simulink model "MPC_simulation"  (R2019b)
settings: Solver=FixedStepDiscrete  StartTime=0.0  StopTime=20  FixedStep=0.01  RelTol=1e-3
InitFcn:
  | Np = 10; Nc = 10;
settings Model: Creator=seokhun  LastModifiedBy=seokhun
settings DebuggingCC: UnderSpecifiedDimensionMsg=warning

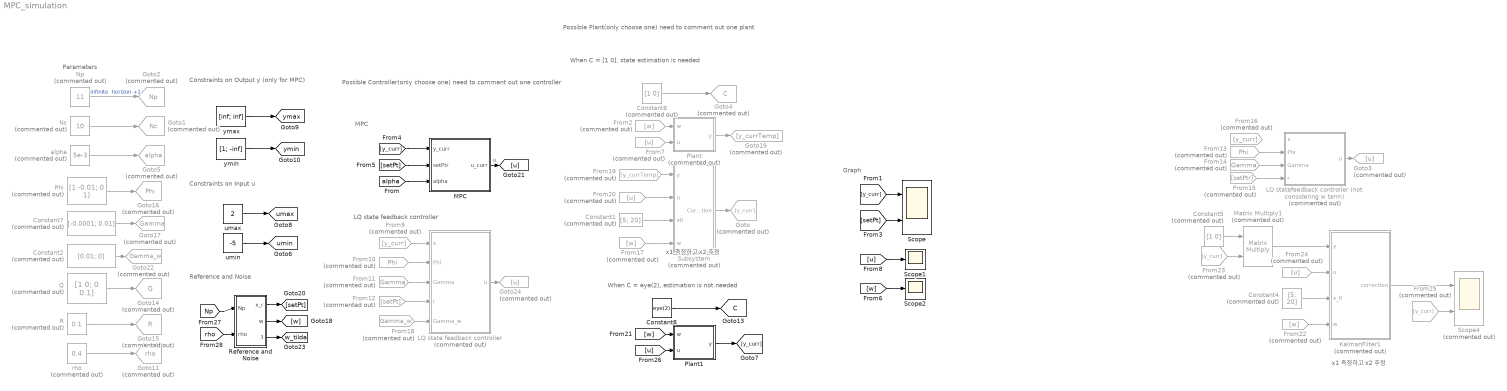
== system MPC_simulation ==
  note: Constraints on Input u
  note: LQ state feedback controller
  note: MPC
  note: Possible Plant(only choose one)
      | need to comment out one plant
  note: When C = eye(2), estimation is not needed
  note: When C = [1 0], state estimation is needed
  note: x1 측정하고 x2 추정
  note: x1 측정하고 x2 추정
  note: Possible Controller(only choose one)
      | need to comment out one controller
  note: Reference and Noise
  note: Parameters
  note: Graph
  note: Constraints on Output y
      | (only for MPC)
  Constant1 : Constant  Commented=on  Value=[5; 20]
  Constant2 : Constant  Commented=on  Value=[0.01; 0]  VectorParams1D=off
  Constant4 : Constant  Commented=on  Value=[5; 20]
  Constant5 : Constant  Commented=on  Value=[1 0]  VectorParams1D=off
  Constant6 : Constant  Commented=on  Value=[1 0]  VectorParams1D=off
  Constant7 : Constant  Commented=on  Value=[-0.0001; 0.01]  VectorParams1D=off
  Constant8 : Constant  Value=eye(2)  VectorParams1D=off
  From10 : From  Commented=on  GotoTag=Phi  TagVisibility=global
  From11 : From  Commented=on  GotoTag=Gamma  TagVisibility=global
  From12 : From  Commented=on  GotoTag=setPt
  From13 : From  Commented=on  GotoTag=Phi  TagVisibility=global
  From14 : From  Commented=on  GotoTag=Gamma  TagVisibility=global
  From15 : From  Commented=on  GotoTag=setPtr
  From{9,16,23,25} (4 alike) : From  Commented=on  GotoTag=y_curr
  From17 : From  Commented=on  GotoTag=w
  From18 : From  Commented=on  GotoTag=Gamma_w  TagVisibility=global
  From19 : From  Commented=on  GotoTag=y_currTemp
  From2 : From  Commented=on  GotoTag=w
  From20 : From  Commented=on  GotoTag=u
  From22 : From  Commented=on  GotoTag=w
  From24 : From  Commented=on  GotoTag=u
  From7 : From  Commented=on  GotoTag=u
  Goto : Goto  Commented=on  GotoTag=y_curr
  Goto1 : Goto  Commented=on  GotoTag=Nc  TagVisibility=global
  Goto11 : Goto  Commented=on  GotoTag=rho  TagVisibility=global
  Goto14 : Goto  Commented=on  GotoTag=Q  TagVisibility=global
  Goto15 : Goto  Commented=on  GotoTag=R  TagVisibility=global
  Goto16 : Goto  Commented=on  GotoTag=Phi  TagVisibility=global
  Goto17 : Goto  Commented=on  GotoTag=Gamma  TagVisibility=global
  Goto19 : Goto  Commented=on  GotoTag=y_currTemp
  Goto2 : Goto  Commented=on  GotoTag=Np  TagVisibility=global
  Goto22 : Goto  Commented=on  GotoTag=Gamma_w  TagVisibility=global
  Goto24 : Goto  Commented=on  GotoTag=u
  Goto3 : Goto  Commented=on  GotoTag=u
  Goto4 : Goto  Commented=on  GotoTag=C  TagVisibility=global
  Goto5 : Goto  Commented=on  GotoTag=alpha  TagVisibility=global
  KalmanFilter1 : MATLAB Function  Commented=on  TreatAsAtomicUnit=on
  LQ state feedback controller : Subsystem  Commented=on
  LQ statefeedback controller (not considering w term) : Subsystem  Commented=on
  MPC : Subsystem
  Matrix Multiply1 : Product  Commented=on  Multiplication=Matrix(*)
  Nc : Constant  Commented=on  Value=10
  Np : Constant  Commented=on  Value=11
  Phi : Constant  Commented=on  Value=[1 -0.01; 0 1]
  Plant : Subsystem  Commented=on
  Plant1 : Subsystem
  Q : Constant  Commented=on  Value=[1 0; 0 0.1]
  R : Constant  Commented=on  Value=0.1  VectorParams1D=off
  Reference and Noise : Subsystem
  Scope : Scope  NumInputPorts=2
  Scope1 : Scope
  Scope2 : Scope
  Scope4 : Scope  Commented=on  NumInputPorts=2
  Subsystem : Subsystem  Commented=on
  alpha : Constant  Commented=on  Value=5e-3
  rho : Constant  Commented=on  Value=0.4
  umax : Constant  Value=2
  umin : Constant  Value=-5
  ymax : Constant  Value=[inf; inf]  VectorParams1D=off
  ymin : Constant  Value=[1; -inf]  VectorParams1D=off
  tag scope: C=global, umax=global, umin=global, w_tilda=global, ymax=global, ymin=global
  wires:
  alpha/1 -> Goto5/1
  Nc/1 -> Goto1/1
  Np/1 -> Goto2/1  "infinite  horizon +1"
  R/1 -> Goto15/1
  Constant8/1 -> [C]
  Phi/1 -> Goto16/1
  Constant7/1 -> Goto17/1
  Q/1 -> Goto14/1
  Reference and Noise/1(x_r) -> [setPt]
  Plant/1(y) -> Goto19/1
  From2/1 -> Plant/1(w)
  [y_curr] -> Scope/1
  [setPt] -> Scope/2
  Reference and Noise/2(w) -> [w]
  [y_curr] -> MPC/1(y_curr)
  [setPt] -> MPC/2(setPtr)
  [alpha] -> MPC/3(alpha)
  [w] -> Scope2/1
  MPC/1(u_curr) -> [u]  "u"
  From7/1 -> Plant/2(u)
  [u] -> Scope1/1
  Constant2/1 -> Goto22/1
  Reference and Noise/3(w_tilda) -> [w_tilda]
  From9/1 -> LQ state feedback controller/1(x)
  From10/1 -> LQ state feedback controller/2(Phi)
  From11/1 -> LQ state feedback controller/3(Gamma)
  From12/1 -> LQ state feedback controller/4(r)
  LQ state feedback controller/1(u) -> Goto24/1
  LQ statefeedback controller (not considering w term)/1(u) -> Goto3/1
  From15/1 -> LQ statefeedback controller (not considering w term)/4(r)
  From14/1 -> LQ statefeedback controller (not considering w term)/3(Gamma)
  From13/1 -> LQ statefeedback controller (not considering w term)/2(Phi)
  From18/1 -> LQ state feedback controller/5(Gamma_w)
  From25/1 -> Scope4/2
  KalmanFilter1/1(correction) -> Scope4/1
  Constant5/1 -> Matrix Multiply1/1
  Matrix Multiply1/1 -> KalmanFilter1/1(y)
  From23/1 -> Matrix Multiply1/2
  From24/1 -> KalmanFilter1/2(u)
  Constant4/1 -> KalmanFilter1/3(x_0)
  From22/1 -> KalmanFilter1/4(w)
  Constant6/1 -> Goto4/1
  [u] -> Plant1/2(u)
  [w] -> Plant1/1(w)
  Plant1/1(y) -> [y_curr]
  From19/1 -> Subsystem/1(y)
  From20/1 -> Subsystem/2(u)
  Constant1/1 -> Subsystem/3(x0)
  From17/1 -> Subsystem/4(w)
  Subsystem/1(Correction) -> Goto/1
  [Np] -> Reference and Noise/1(Np)
  umax/1 -> [umax]
  umin/1 -> [umin]
  ymax/1 -> [ymax]
  ymin/1 -> [ymin]
  [rho] -> Reference and Noise/2(rho)
  rho/1 -> Goto11/1

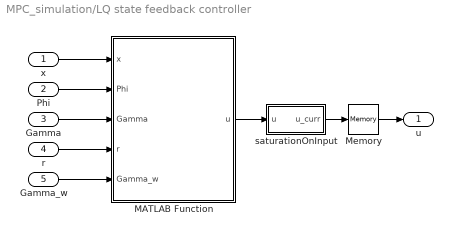
== system MPC_simulation/LQ state feedback controller ==
  x : Inport
  Phi : Inport  Port=2
  Gamma : Inport  Port=3
  r : Inport  Port=4
  Gamma_w : Inport  Port=5
  MATLAB Function : MATLAB Function  TreatAsAtomicUnit=on
  Memory : Memory
  saturationOnInput : Subsystem
  u : Outport
  wires:
  x/1 -> MATLAB Function/1(x)
  saturationOnInput/1(u_curr) -> Memory/1
  Gamma/1 -> MATLAB Function/3(Gamma)
  Memory/1 -> u/1
  r/1 -> MATLAB Function/4(r)
  Phi/1 -> MATLAB Function/2(Phi)
  Gamma_w/1 -> MATLAB Function/5(Gamma_w)
  MATLAB Function/1(u) -> saturationOnInput/1(u)

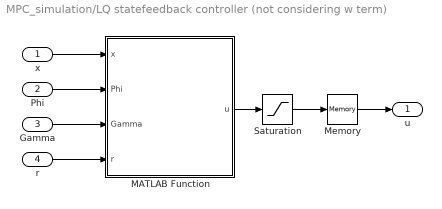
== system MPC_simulation/LQ statefeedback controller (not considering w term) ==
  x : Inport
  Phi : Inport  Port=2
  Gamma : Inport  Port=3
  r : Inport  Port=4
  MATLAB Function : MATLAB Function  TreatAsAtomicUnit=on
  Memory : Memory
  Saturation : Saturate  UpperLimit=2  LowerLimit=-5
  u : Outport
  wires:
  Phi/1 -> MATLAB Function/2(Phi)
  r/1 -> MATLAB Function/4(r)
  Memory/1 -> u/1
  Gamma/1 -> MATLAB Function/3(Gamma)
  Saturation/1 -> Memory/1
  MATLAB Function/1(u) -> Saturation/1
  x/1 -> MATLAB Function/1(x)

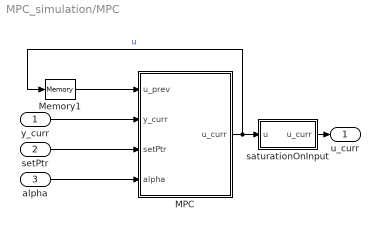
== system MPC_simulation/MPC ==
  y_curr : Inport
  setPtr : Inport  Port=2
  alpha : Inport  Port=3
  MPC : Subsystem
  Memory1 : Memory
  saturationOnInput : Subsystem
  u_curr : Outport
  wires:
  MPC/1(u_curr) -> saturationOnInput/1(u), Memory1/1  "u"
  y_curr/1 -> MPC/2(y_curr)
  alpha/1 -> MPC/4(alpha)
  Memory1/1 -> MPC/1(u_prev)
  setPtr/1 -> MPC/3(setPtr)
  saturationOnInput/1(u_curr) -> u_curr/1

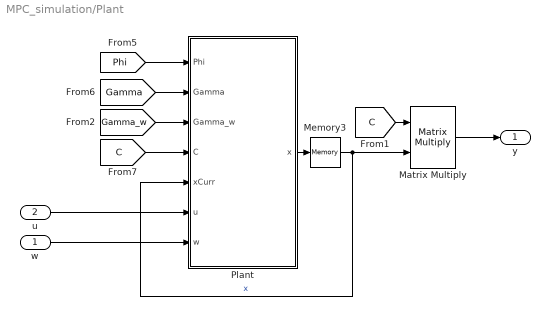
== system MPC_simulation/Plant ==
  w : Inport
  u : Inport  Port=2
  Matrix Multiply : Product  Multiplication=Matrix(*)
  Memory3 : Memory  InitialCondition=[5; 20]
  Plant : MATLAB Function  TreatAsAtomicUnit=on
  y : Outport
  wires:
  Memory3/1 -> Plant/5(xCurr), Matrix Multiply/2  "x"
  u/1 -> Plant/6(u)
  [Gamma] -> Plant/2(Gamma)
  w/1 -> Plant/7(w)
  Plant/1(x) -> Memory3/1
  [C] -> Matrix Multiply/1
  [Phi] -> Plant/1(Phi)
  [C] -> Plant/4(C)
  Matrix Multiply/1 -> y/1
  [Gamma_w] -> Plant/3(Gamma_w)

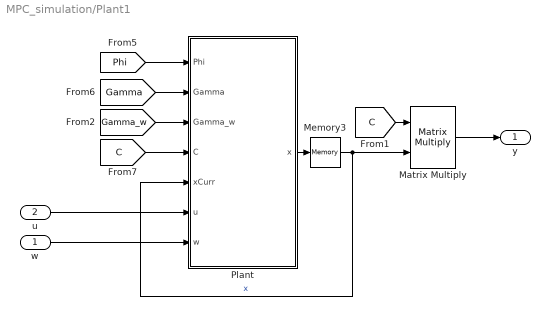
== system MPC_simulation/Plant1 ==
  w : Inport
  u : Inport  Port=2
  Matrix Multiply : Product  Multiplication=Matrix(*)
  Memory3 : Memory  InitialCondition=[5; 20]
  Plant : MATLAB Function  TreatAsAtomicUnit=on
  y : Outport
  wires:
  [Gamma_w] -> Plant/3(Gamma_w)
  Matrix Multiply/1 -> y/1
  [C] -> Plant/4(C)
  [Phi] -> Plant/1(Phi)
  [C] -> Matrix Multiply/1
  Plant/1(x) -> Memory3/1
  w/1 -> Plant/7(w)
  [Gamma] -> Plant/2(Gamma)
  u/1 -> Plant/6(u)
  Memory3/1 -> Matrix Multiply/2, Plant/5(xCurr)  "x"

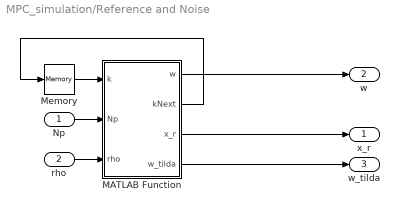
== system MPC_simulation/Reference and Noise ==
  Np : Inport
  rho : Inport  Port=2
  MATLAB Function : MATLAB Function  TreatAsAtomicUnit=on
  Memory : Memory
  x_r : Outport
  w : Outport  Port=2
  w_tilda : Outport  Port=3
  wires:
  MATLAB Function/2(kNext) -> Memory/1
  Memory/1 -> MATLAB Function/1(k)
  MATLAB Function/3(x_r) -> x_r/1
  MATLAB Function/1(w) -> w/1
  MATLAB Function/4(w_tilda) -> w_tilda/1
  Np/1 -> MATLAB Function/2(Np)
  rho/1 -> MATLAB Function/3(rho)

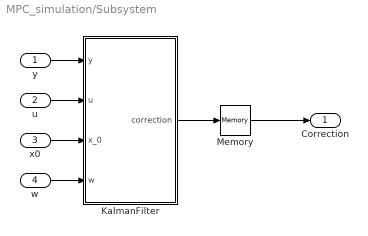
== system MPC_simulation/Subsystem ==
  y : Inport
  u : Inport  Port=2
  x0 : Inport  Port=3
  w : Inport  Port=4
  KalmanFilter : MATLAB Function  TreatAsAtomicUnit=on
  Memory : Memory  InitialCondition=[5; 20]
  Correction : Outport
  wires:
  KalmanFilter/1(correction) -> Memory/1
  x0/1 -> KalmanFilter/3(x_0)
  u/1 -> KalmanFilter/2(u)
  w/1 -> KalmanFilter/4(w)
  y/1 -> KalmanFilter/1(y)
  Memory/1 -> Correction/1

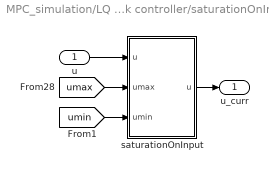
== system MPC_simulation/LQ state feedback controller/saturationOnInput ==
  u : Inport
  saturationOnInput : MATLAB Function  TreatAsAtomicUnit=on
  u_curr : Outport
  wires:
  u/1 -> saturationOnInput/1("u ")
  saturationOnInput/1(u) -> u_curr/1
  [umax] -> saturationOnInput/2(umax)
  [umin] -> saturationOnInput/3(umin)

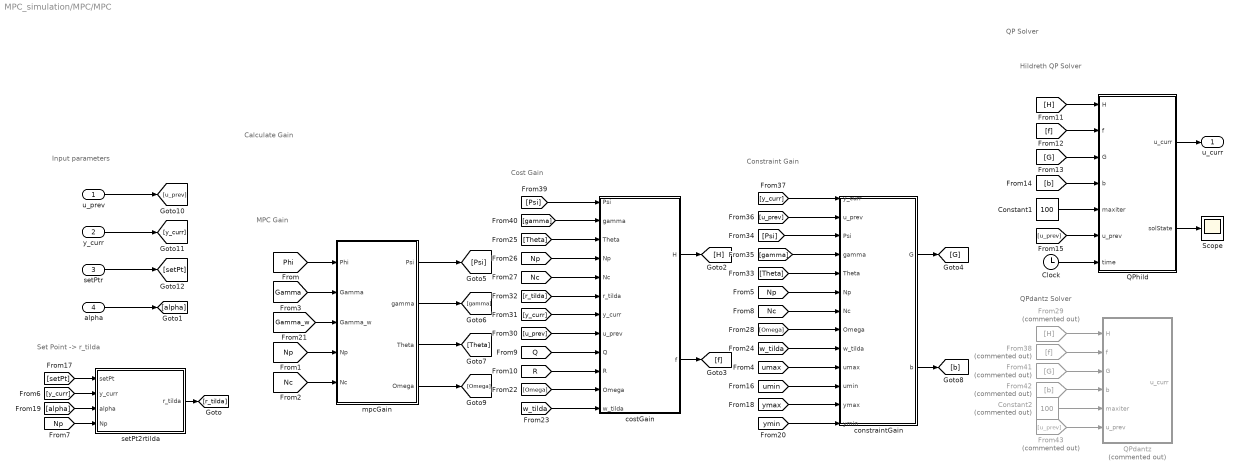
== system MPC_simulation/MPC/MPC ==
  note: QPdantz Solver
  note: Hildreth QP Solver
  note: QP Solver
  note: Set Point -> r_tilda
  note: Cost Gain
  note: Constraint Gain
  note: MPC Gain
  note: Calculate Gain
  note: Input parameters
  u_prev : Inport
  y_curr : Inport  Port=2
  setPtr : Inport  Port=3
  alpha : Inport  Port=4
  Clock : Clock
  Constant1 : Constant  Value=100
  Constant2 : Constant  Commented=on  Value=100
  From29 : From  Commented=on  GotoTag=H
  From38 : From  Commented=on  GotoTag=f
  From41 : From  Commented=on  GotoTag=G
  From42 : From  Commented=on  GotoTag=b
  From43 : From  Commented=on  GotoTag=u_prev
  QPdantz : MATLAB Function  Commented=on  TreatAsAtomicUnit=on
  QPhild : MATLAB Function  TreatAsAtomicUnit=on
  Scope : Scope
  constraintGain : MATLAB Function  TreatAsAtomicUnit=on
  costGain : MATLAB Function  TreatAsAtomicUnit=on
  mpcGain : MATLAB Function  TreatAsAtomicUnit=on
  setPt2rtilda : MATLAB Function  TreatAsAtomicUnit=on
  u_curr : Outport
  wires:
  [Phi] -> mpcGain/1(Phi)
  [Np] -> mpcGain/4(Np)
  mpcGain/1(Psi) -> [Psi]
  [setPt] -> setPt2rtilda/1(setPt)
  u_prev/1 -> [u_prev]
  [Gamma] -> mpcGain/2(Gamma)
  mpcGain/3(Theta) -> [Theta]
  mpcGain/2(gamma) -> [gamma]
  setPtr/1 -> [setPt]
  y_curr/1 -> [y_curr]
  setPt2rtilda/1(r_tilda) -> [r_tilda]
  [y_curr] -> setPt2rtilda/2(y_curr)
  [Np] -> setPt2rtilda/4(Np)
  [alpha] -> setPt2rtilda/3(alpha)
  alpha/1 -> [alpha]
  [Nc] -> mpcGain/5(Nc)
  [Psi] -> constraintGain/3(Psi)
  [u_prev] -> constraintGain/2(u_prev)
  [y_curr] -> constraintGain/1(y_curr)
  [Theta] -> constraintGain/5(Theta)
  [gamma] -> constraintGain/4(gamma)
  [r_tilda] -> costGain/6(r_tilda)
  [u_prev] -> costGain/8(u_prev)
  [Psi] -> costGain/1(Psi)
  [Np] -> costGain/4(Np)
  [y_curr] -> costGain/7(y_curr)
  [Theta] -> costGain/3(Theta)
  [gamma] -> costGain/2(gamma)
  Constant1/1 -> QPhild/5(maxiter)
  [Nc] -> costGain/5(Nc)
  [Np] -> constraintGain/6(Np)
  [Nc] -> constraintGain/7(Nc)
  [Q] -> costGain/9(Q)
  [R] -> costGain/10(R)
  costGain/1(H) -> [H]
  costGain/2(f) -> [f]
  constraintGain/1(G) -> [G]
  constraintGain/2(b) -> [b]
  [H] -> QPhild/1(H)
  [f] -> QPhild/2(f)
  [G] -> QPhild/3(G)
  [b] -> QPhild/4(b)
  [u_prev] -> QPhild/6(u_prev)
  [Gamma_w] -> mpcGain/3(Gamma_w)
  mpcGain/4(Omega) -> [Omega]
  [Omega] -> costGain/11(Omega)
  [w_tilda] -> costGain/12(w_tilda)
  [w_tilda] -> constraintGain/9(w_tilda)
  [Omega] -> constraintGain/8(Omega)
  From42/1 -> QPdantz/4(b)
  From41/1 -> QPdantz/3(G)
  From38/1 -> QPdantz/2(f)
  From29/1 -> QPdantz/1(H)
  Constant2/1 -> QPdantz/5(maxiter)
  From43/1 -> QPdantz/6(u_prev)
  QPhild/1(u_curr) -> u_curr/1
  Clock/1 -> QPhild/7(time)
  QPhild/2(solState) -> Scope/1
  [umax] -> constraintGain/10(umax)
  [umin] -> constraintGain/11(umin)
  [ymax] -> constraintGain/12(ymax)
  [ymin] -> constraintGain/13(ymin)

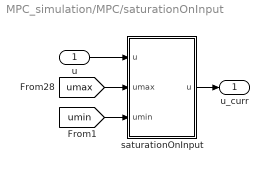
== system MPC_simulation/MPC/saturationOnInput ==
  u : Inport
  saturationOnInput : MATLAB Function  TreatAsAtomicUnit=on
  u_curr : Outport
  wires:
  u/1 -> saturationOnInput/1("u ")
  saturationOnInput/1(u) -> u_curr/1
  [umax] -> saturationOnInput/2(umax)
  [umin] -> saturationOnInput/3(umin)

== matlab function MPC_simulation/MPC/MPC/mpcGain ==
  data: Phi input; Psi output; Gamma input; Gamma_w input; Np input; gamma output; Theta output; Nc input; Omega output
function [Psi, gamma, Theta, Omega] = mpcGain(Phi, Gamma, Gamma_w, Np, Nc)
%%% x(k+1) = Phi*x(k) + Gamma*u(k)
%%% y(k) = C*x(k)

persistent first Psi_y gamma_y Theta_y Omega_y

% Np = 21; Nc = 10;
Np = 11; Nc = 10;
if isempty(first)
    C = eye(2);
    first = 1;    
    %%%%% Find Psi_x, gamma_x, Theta_x and Omega_x
    %%% Psi_x
    [nx, ~] = size(Phi);
    Psi_x = zeros(nx*Np, nx);
    Psi_x(1:nx, :) = eye(nx);
    for i=2:Np    
        Psi_x(nx*(i-1)+1:nx*i, :) = Psi_x(nx*(i-2)+1:nx*(i-1), :)*Phi;
    end

    %%% gamma_x
    [~, nu] = size(Gamma);
    gamma_x = zeros(nx*Np, nu);
    temp = Gamma;
    tempSum = Gamma;
    for i=2:Np
        gamma_x(nx*(i-1)+1:nx*i, :) = tempSum;
        temp = Phi*temp;
        tempSum = tempSum + temp;
    end

    % gamma_xx = [zeros(nx,nu); Gamma; Phi*Gamma+Gamma; Phi^2*Gamma+Phi*Gamma+Gamma]

    %%% Theta_x
    Theta_x = zeros(nx*Np, nu*Nc);
    for j=1:Nc
        if nu == 1
            Theta_x(nx*(j-1)+1:end, j) = gamma_x(1:nx*Np-nx*(j-1), :);
        else
           Theta_x(nx*(j-1)+1:end, nu*(j-1)+1:nu*j) = gamma_x(1:nx*Np-nx*(j-1), :);
        end
    end
    
    %%% Omega_x
    [~, nw] = size(Gamma_w);
    Omega_x = zeros(nx*Np, nw*Np);
    vec = zeros(nx*Np, nw);
    for i=2:Np
        vec(nx*(i-1)+1:nx*i, :) = Psi_x(nx*(i-2)+1:nx*(i-1), :)*Gamma_w;
    end
    for i=1:Np
        if nw == 1
            Omega_x(nx*(i-1)+1:end, i) = vec(1:nx*Np-nx*(i-1), :);
        else        
            Omega_x(nx*(i-1)+1:end, nw*(i-1)+1:nw*i) = vec(1:nx*Np-nx*(i-1), :);
        end
    end
    
    %%%%% Find Psi_x, gamma_x, Theta_x and Omega_x

    %%%%% Find Psi_y, gamma_y, Theta_y and Omega_y
    %%%%% which is equal Psi, gamma, Theta and Omega respectively
    [ny, ~] = size(C);
    C_tilda = zeros(ny*Np, nx*Np);
    for i=1:Np
        if ny == 1            
            C_tilda(i, nx*(i-1)+1:nx*i) = C;
        else
            C_tilda(ny*(i-1)+1:ny*i, nx*(i-1)+1:nx*i) = C;
        end
    end
    Psi_y = C_tilda*Psi_x*C'*(C*C')^-1;
    gamma_y = C_tilda*gamma_x;
    Theta_y = C_tilda*Theta_x;    
    Omega_y = C_tilda*Omega_x;
    %%%%% Find Psi_y, gamma_y, Theta_y and Omega_y
    %%%%% which is equal Psi, gamma, Theta and Omega respectively
end

Psi = Psi_y;
gamma = gamma_y;
Theta = Theta_y;
Omega = Omega_y;

== matlab function MPC_simulation/Plant/Plant ==
  data: Phi input; Gamma input; Gamma_w input; C input; xCurr input; u input; x output; w input
function x  = plant(Phi, Gamma, Gamma_w, C, xCurr, u, w)
% Phi = [1 0.01; 0 1];
% Gamma = [-0.0001; -0.01];
% C = eye(2);

% xNext = Phi*xCurr + Gamma*u; % x(k+1) = Phi*x(k) + gamma2*u(k)
xNext = Phi*xCurr + Gamma*u + Gamma_w*w; % x(k+1) = Phi*x(k) + gamma2*u(k)
x = xNext;
end

== matlab function MPC_simulation/LQ state feedback controller/MATLAB Function ==
  data: x input; Phi input; Gamma input; r input; Gamma_w input; u output
function u = LQcontroller(x, Phi, Gamma, r, Gamma_w)
persistent first leftInv a b nx 
if isempty(first)
    first = 1;
    a = 1; b = 0.1;
    Czx = [a 0; 0 b]; Dzu = [0; 0];
    A = [eye(2)-Phi Gamma; -Czx Dzu];
    [nx, ~] = size(Phi);
    leftInv = (A'*A)^-1*A';
%     xeq = zeros(nx,1); xeq(:) = -p(1:nx); 
%     ueq = zeros(size(Gamma,2)); ueq(:) = p(nx+1:end);
end

% a = 1;  b = 0.1; Czx = [a 0; 0 b];
% Dzu = [0; 0];
% rho = 0.1;
% Q = Czx'*Czx; R = Dzu'*Dzu+rho; N = Czx'*Dzu;
% Phi = [1 -0.01; 0 1]; Gamma = [-0.0001; 0.01];
% [K, ~, ~] = dlqr(Phi, Gamma, Q, R, N);
K = [-3.122453376782691,2.502849098184925];

r(1) = r(1)*a; r(2) = r(2)*b;
w = 20;
q = [-Gamma_w*w; r];
p = leftInv*q; % Ap = q

xeq = zeros(nx,1); xeq(:) = -p(1:nx);
ueq = zeros(size(Gamma,2)); ueq(:) = p(nx+1:end);
u = zeros(size(Gamma,2));
u(:) = -K*(x-xeq) + ueq;
end

== matlab function MPC_simulation/LQ statefeedback controller (not considering w term)/MATLAB Function ==
  data: x input; u output; Phi input; Gamma input; r input
function u = LQcontroller(x, Phi, Gamma, r)
persistent first leftInv a b nx 
if isempty(first)
    first = 1;
    a = 1; b = 0.1;
    Czx = [a 0; 0 b]; Dzu = [0; 0];
    A = [eye(2)-Phi Gamma; -Czx Dzu];
    [nx, ~] = size(Phi);
    leftInv = (A'*A)^-1*A';
end

r(1) = r(1)*a; r(2) = r(2)*b;

q = [zeros(nx,1); r];
p = leftInv*q; % Ap = q 
xeq = zeros(nx,1); xeq(:) = -p(1:nx); 
ueq = zeros(size(Gamma,2)); ueq(:) = p(nx+1:end);

% a = 1;  b = 0.1; G = [a 0; 0 b];
% H = [0; 0];
% rho = 0.1;
% Q = G'*G; R = H'*H+rho; N = G'*H;
% Phi = [1 -0.01; 0 1]; Gamma = [-0.0001; 0.01];
% [K, ~, ~] = dlqr(Phi, Gamma, Q, R, N);
K = [-3.122453376782691,2.502849098184925];


u = zeros(size(Gamma,2));
u(:) = -K*(x-xeq) + ueq;
end

== matlab function MPC_simulation/MPC/MPC/setPt2rtilda ==
  data: setPt input; r_tilda output; y_curr input; alpha input; Np input
function r_tilda = set_pt2r_tilda(setPt, y_curr, alpha, Np)
%%% r_tilda = y_r_tilda(set-point) + r_e_tilda
%%% where r_e(k+i) = y_e(k)*exp(-alpha*i)

Np = 11;
% Np = 21;
[ny, ~] = size(y_curr);
r_tilda = zeros(ny*Np,1);

y_e = y_curr - setPt;

for i=1:Np
    r_tilda(ny*(i-1)+1:ny*i) = setPt + y_e * exp(-alpha*(i-1));
end

== matlab function MPC_simulation/Reference and Noise/MATLAB Function ==
  data: k input; w output; kNext output; x_r output; w_tilda output; Np input; rho input
function [w, kNext, x_r, w_tilda] = makeNoise(k, Np, rho)

delta_k = 25;

x1_r = 5;
x2_r = noise(max(1, k-delta_k), rho);
x_r = [x1_r; x2_r];

w = noise(k, rho);

w_tilda = make_w_tilda(k, Np, rho);

kNext = k + 1;

end

function w = noise(k, rho)

% rho = 0.4;
w0 = 20; ks = 500; kf = ks + 200; 
w = w0*(1-rho*(sin(pi*(min(max(0,k-ks),kf-ks)/(kf-ks)))^2));

end

function w_tilda = make_w_tilda(k, Np, rho)
Np = 11; %%%%%%%%%%%%%%%%%%%%%%
% Np = 21; %%%%%%%%%%%%%%%%%%%%%%
w_tilda = zeros(Np,1);
for i=1:Np
    w_tilda(i) = noise(k+i-1, rho);
end
end

== matlab function MPC_simulation/MPC/MPC/QPdantz ==
  data: H input size=[10, 10]; u_curr output size=1; f input size=[10, 1]; G input size=[84, 10]; b input size=[84, 1]; maxiter input size=1; u_prev input size=1
function u_curr = QPdantzSolver(H, f, G, b, maxiter, u_prev)
nx = 2; Np = 11;
Nc = 10; nu = 1;

delta_u_tilda_umin = -5*ones(nu*Nc,1);

delta_u_tilda = zeros(Nc*nu, 1);
[delta_u_tilda(:), ~, ~] = qpdantzMy(H, f, G, b, delta_u_tilda_umin, maxiter);
% [delta_u_tilda(:), ~, ~] = quadprog(H, f, G, b);

u_curr = zeros(nu,1); 
u_curr(:) = delta_u_tilda(1) + u_prev;
end


function [xopt,lambda,how] = qpdantzMy(H,f,A,b,xmin,maxiter)
%QPDANTZ command will be removed in a future release.  If you have
%   Optimization Toolbox, replace "qpdantz" with "quadprog" command. 
%
% QPDANTZ solves a quadratic program using an active set method.
%
%   [x,lambda,status]=QPDANTZ(H,f,A,b,xmin,maxiter) solves the quadratic
%   programming problem:
%
%     min 0.5*x'Hx + f'x   subject to:  Ax <= b, x >= xmin
%      x
%
%   where:
%        x = the optimal solution vector.
%   lambda = the dual variables (Lagrange multipliers) at the solution.
%   status = 'feasible' if x satisfies the constraints
%          = 'infeasible' if no feasible x could be found
%          = 'unreliable' if maximum number of iterations is exceeded.

%   Author: A. Bemporad
%   Copyright 1986-2011 The MathWorks, Inc.

narginchk(4,6);

if nargin<5 || isempty(xmin)
    xmin=-1e3*ones(size(f(:)));
%     ctrlMsgUtils.warning('MPC:computation:AssumeXMin');    
end

if nargin<6,
    maxiter=200;
end
if maxiter<1,
%     ctrlMsgUtils.error('MPC:computation:InvalidMAXITER','qpdantz');
end

mnu=length(f);
nc=length(b);

if ~isequal(size(H),[mnu mnu])
%     ctrlMsgUtils.error('MPC:computation:InvalidHessianOrLinCost','qpdantz');            
end

if size(A,2)~=mnu,
%     ctrlMsgUtils.error('MPC:computation:InvalidConsMatrixOrLinCost','qpdantz');                
end

if size(A,1)~=nc,
%     ctrlMsgUtils.error('MPC:computation:InvalidConsMatrixOrRHS','qpdantz');                
end

% H must be symmetric. Otherwise set H=(H+H')/2
if norm(H-H') > eps
%     ctrlMsgUtils.warning('MPC:computation:HessianNonsymmetric');    
    H = (H+H')*0.5;
end

% Force double precision
xmin=double(xmin);
H=double(H);
f=double(f);
A=double(A);
b=double(b);
maxiter=double(maxiter);

% This is a constant term that adds to the initial basis in each QP.
% sw=ctrlMsgUtils.SuspendWarnings;
a=-H*xmin(:);    
% Inverted hessian
H=H\eye(mnu);
% delete(sw);
rhsc=b(:)-A*xmin(:);
rhsa=a-f(:);
TAB=[-H H*A';A*H -A*H*A'];
basisi=[H*rhsa;
    rhsc-A*H*rhsa];
ibi=-(1:mnu+nc)';
ili=-ibi;
[basis,ib,il,iter] = qpdantzg(TAB,basisi,ibi,ili,maxiter);

if iter>maxiter,
    how='unreliable';
elseif iter <=0
    how='infeasible';    
else
    how='feasible';
end

xopt=zeros(mnu,1);

for j=1:mnu
    if il(j) <= 0
        xopt(j)=xmin(j);
    else
        xopt(j)=basis(il(j))+xmin(j);
    end
end

% Add additonal check to avoild numerical issues in QPDANTZG
if any((A*xopt-b)>sqrt(eps)*abs(b))
    how='infeasible';    
end

if nargout>=2,
    lambda=zeros(nc,1);
    for j=1:nc,
        if ib(mnu+j) <= 0
            lambda(j)=0;
        else
            lambda(j)=basis(ib(mnu+j));
        end
    end
end

% ctrlMsgUtils.warning('MPC:utility:ObsoleteQPdantz');    
end

== matlab function MPC_simulation/MPC/MPC/costGain ==
  data: Psi input; H output; gamma input; Theta input; Np input; Nc input; r_tilda input; y_curr input; u_prev input; f output; Q input; R input; Omega input; w_tilda input
function [H, f] = costGain(Psi, gamma, Theta, Np, Nc, r_tilda, y_curr, u_prev, ...
   Q, R, Omega, w_tilda)

Np = Np-1; %%%%%%%%% for infinite horizon MPC

%%%%% Find QP problem parameters H and f
%%%%% 0.5*detla_u_tilda'*H*detla_u_tilda + detla_u_tilda'*f + fo
%%%%% where z(k) = Czy*(y(k)-r(k)) + Dzu*delta_u(k)
%%%%% and J_N = (y_tilda(k)-r_tilda(k))'*Q_tilda*(y_tilda(k)-r_tilda(k))
%%%%% + u_tilda(k)'*R_tilda*u_tilda(k)
Nc = 10;
persistent first Hsaved Q_tilda R_tilda Q_bar
if isempty(first)
    C = eye(2);
    first = 1;
    [ny, ~] = size(y_curr);
    Q_tilda = zeros(ny*Np, ny*Np);
    for i=1:Np
        if ny == 1            
            Q_tilda(i, i) = Q;
        else
            Q_tilda(ny*(i-1)+1:ny*i, ny*(i-1)+1:ny*i) = Q;
        end
    end

    [nu, ~] = size(u_prev);    
    R_tilda = zeros(nu*Nc, nu*Nc);
    for i=1:Nc
        if nu == 1            
            R_tilda(i, i) = R;
        else
            R_tilda(nu*(i-1)+1:nu*i, nu*(i-1)+1:nu*i) = R;
        end
    end
    
    %%%% infinite horizon %%%%
    
%     [P_bar, ~, ~] = idare(Phi, Gamma, Q, R);
    P_bar = [85.586998992535270,-31.197736987778430;
        -31.197736987778430,26.801206841423674];
    P_bar_y = (C*C')^-1*C*P_bar*C'*(C*C')^-1;
    Q_bar = blkdiag(Q_tilda, P_bar_y);
    
    Hsaved = 2*(Theta'*Q_bar*Theta + R_tilda);
    
    %%%% infinite horizon %%%%
    
%     Hsaved = 2*(Theta'*Q_tilda*Theta + R_tilda);  %%%% finite horizon %%%%
end

%%% r_tilda = y_r_tilda(set-point) + r_e_tilda
%%% where r_e(k+i) = y_e(k)*exp(-alpha*i)
c_tilda = r_tilda - Psi*y_curr - gamma*u_prev;
[nu, ~] = size(u_prev);
f = zeros(nu*Nc,1);
% f(:) = -2*Theta'*Q_tilda*(c_tilda - Omega*w_tilda);  %%%% finite horizon %%%%
f(:) = -2*Theta'*Q_bar*(c_tilda - Omega*w_tilda);  %%%% infinite horizon %%%%
H = Hsaved;

== matlab function MPC_simulation/MPC/MPC/QPhild ==
  data: H input; u_curr output; f input; G input; b input; maxiter input; u_prev input; time input; solState output
function [u_curr, solState] = QPhild(H, f, G, b, maxiter, u_prev, time)
%%% minimize J = 0.5*x'*H*x + f'*x 
%%% s.t Gx <= b
[nb, ~] = size(G); 
delta_u_tilda = -H^-1*f; 
solState = 0;
%%% Whether it is unconstrained problem
kk = 0;
for i=1:nb
    if (G(i,:)*delta_u_tilda > b(i)) 
        kk = kk + 1;
    else
        kk = kk + 0;
    end
end
if (kk==0)
%     fprintf("unconstrained problem at t = %f\n", time);
    u_curr = delta_u_tilda(1) + u_prev;
    solState = 1;
    return;
end
%%% Whether it is unconstrained problem

H_bar = G*H^-1*G';

f_bar = G*H^-1*f + b;
[nb, m] = size(f_bar);
lambda = zeros(nb, m);
for km=1:maxiter
    % find the elements in the solution vector one by one
    % km could be larger if the Lagranger multiplier has a slow
    % convergence rate.
    lambda_prev = lambda;
    for i=1:nb
        w = H_bar(i,:)*lambda - H_bar(i,i)*lambda(i,1) + f_bar(i,1);
        la = -w/H_bar(i,i);
        lambda(i,1)=max(0,la);
    end
    al = (lambda-lambda_prev)'*(lambda-lambda_prev);
    if (al<1e-14)
%         fprintf("constrained problem at t = %f\n", time);
        solState = 2;
        break;
    end    
end

if (km == maxiter)
%     fprintf("no feasible at t = %f\n", time);
    solState = 3;
end

delta_u_tilda = -H^-1*(f + G'*lambda);

u_curr = delta_u_tilda(1) + u_prev;

end

== matlab function MPC_simulation/MPC/MPC/constraintGain ==
  data: y_curr input; G output; u_prev input; Psi input; gamma input; Theta input; b output; Np input; Nc input; Omega input; w_tilda input; umax input; umin input; ymax input; ymin input
function [G, b] = constraintGain(y_curr, u_prev, Psi, gamma, Theta, Np, Nc, ...
    Omega, w_tilda, umax, umin, ymax, ymin)

% Np = 21; Nc = 10; %%%%%%%%%%%%%%%%%%%%%%%%%%%%%%%%%%%%%%%%%%
Np = 11; Nc = 10; %%%%%%%%%%%%%%%%%%%%%%%%%%%%%%%%%%%%%%%%%%

%%%%%% constraint on y %%%%%%
% ymin = [1; -inf]; ymax = [7; 21.5]; %%%%%%%%%%%%%%%%%%%%%%%%%%%%%%%%%%%%%%%%%%
% ymin = [1; -inf]; ymax = [inf; inf]; %%%%%%%%%%%%%%%%%%%%%%%%%%%%%%%%%%%%%%%%%%
[ny, ~] = size(y_curr);
Gy = [-eye(Np*ny); eye(Np*ny)];
gy = zeros(Np*ny*2,1);
for i=1:Np
    gy(ny*(i-1)+1:ny*i) = -ymin;
    gy(ny*(i-1)+1+Np*ny:ny*i+Np*ny) = ymax;
end
  
%%%%%% constraint on u %%%%%%
[nu, ~] = size(u_prev);
C1 = ones(Nc,1); 
Fo = [-C1; C1];
vec = ones(Nc,1); C2 = zeros(Nc,Nc); 
C2(:,1) = vec; % first column of C2
for i=2:Nc
    C2(:,i)=[zeros((i-1),1);vec(1:(Nc-i+1),1)]; 
end
Fd = [-C2; C2];
% umin = -2; umax = 1; %%%%%%%%%%%%%%%%%%%%%%%%%%%%%%%%%%%%%%%%%%
% umin = -5; umax = 2; %%%%%%%%%%%%%%%%%%%%%%%%%%%%%%%%%%%%%%%%%%
gu = [-umin*ones(Nc,1); umax*ones(Nc,1)];

%%%%%% constraint on delta_u %%%%%%
Gdeltau = [-eye(Nc); eye(Nc)];
deltau_min = -inf; deltau_max = inf; %%%%%%%%%%%%%%%%%%%%%%%%%%%%%%%%%%%%%%%%%%
% deltau_min = -1; deltau_max = 1; %%%%%%%%%%%%%%%%%%%%%%%%%%%%%%%%%%%%%%%%%%
gdeltau = [-deltau_min*ones(Nc,1); deltau_max*ones(Nc,1)];

G = [Gy*Theta; Fd; Gdeltau];
bo = [gy - Gy*Omega*w_tilda; gu; gdeltau]; %%%%%%%%%%%%% << disturbance considering model
% bo = [gy; gu; gdeltau]; %%%%%%%%%%%%% << no dsturbance model
Bp = [-Gy*Psi -Gy*gamma; zeros(size(Fd,1), ny) -Fo; zeros(size(Gdeltau,1),ny+nu)]; 
p = [y_curr; u_prev];
b = bo + Bp*p;

== matlab function MPC_simulation/KalmanFilter1 ==
  data: y input; u input; correction output; x_0 input; w input
function correction = KalmanFilter(y, u, x_0, w)
persistent first
persistent Phi Gamma Gamma_w C D Q R P x 

if isempty(first)
    first = 1;
    Phi = [1 -0.01; 0 1];
    Gamma = [-0.0001; 0.01];
    Gamma_w = [0.01; 0];
%     C = [1 0];
    C = [1 0];
    D = zeros(2,1);
    Q = 0.5*eye(2); R = 0.01;
    P = 2*eye(2);
    x = x_0; 
end


xp = Phi*x + Gamma*u + Gamma_w*w;
% Pp = Phi*P*Phi' + Q;
Pp = Phi*P*Phi' - Phi*P*C'*(C*P*C'+R)^-1*C*P*Phi' + Q;
K = Pp*C'*(C*Pp*C' + R)^-1;
x = xp + K*(y - C*xp);
P = (eye(2)-K*C)*Pp;

correction = x;
end

== matlab function MPC_simulation/Plant1/Plant ==
  data: Phi input; Gamma input; Gamma_w input; C input; xCurr input; u input; x output; w input
function x  = plant(Phi, Gamma, Gamma_w, C, xCurr, u, w)
% Phi = [1 0.01; 0 1];
% Gamma = [-0.0001; -0.01];
% C = eye(2);

% xNext = Phi*xCurr + Gamma*u; % x(k+1) = Phi*x(k) + gamma2*u(k)
xNext = Phi*xCurr + Gamma*u + Gamma_w*w; % x(k+1) = Phi*x(k) + gamma2*u(k)
x = xNext;
end

== matlab function MPC_simulation/MPC/saturationOnInput/saturationOnInput ==
  data: u input; u output; umax input; umin input
function u = fcn(u, umax, umin)
if u > umax
    u = umax;
elseif u < umin 
    u = umin;
end
end

== matlab function MPC_simulation/LQ state feedback controller/saturationOnInput/saturationOnInput ==
  data: u input; u output; umax input; umin input
function u = fcn(u, umax, umin)
if u > umax
    u = umax;
elseif u < umin 
    u = umin;
end
end

== matlab function MPC_simulation/Subsystem/KalmanFilter ==
  data: y input; u input; correction output size=[2;1]; x_0 input; w input
function correction = KalmanFilter(y, u, x_0, w)
persistent first
persistent Phi Gamma Gamma_w C Q R P x 

if isempty(first)
    first = 1;
    Phi = [1 -0.01; 0 1];
    Gamma = [-0.0001; 0.01];
    Gamma_w = [0.01; 0];
    C = [1 0];
%     Q = 0.5*eye(2); R = 0.01;
%     P = 2*eye(2);
    Q = 20*eye(2); R = 0.01;
    P = 0.1*eye(2);
    x = x_0; 
end


% xp = Phi*x + Gamma*u;
xp = Phi*x + Gamma*u + Gamma_w*w;
Pp = Phi*P*Phi' - Phi*P*C'*(C*P*C'+R)^-1*C*P*Phi' + Q;
K = Pp*C'*(C*Pp*C' + R)^-1;
x = xp + K*(y - C*xp);
P = (eye(2)-K*C)*Pp;

correction = x;
end
